simulink model "Non_linear_simulation"  (R2020b)
settings: Solver=FixedStepAuto  StartTime=0.0  StopTime=10  FixedStep=.001  RelTol=1e-3  EnableMultiTasking=on
values from neighbouring files (symbols this model uses):
  alphaPlotHandle = plot(inf,inf,'-b','linewidth',2)    [initialiseVisualiser.m]
  armPartPatchHandle = patch(Xt,Yt,Zt,C,'Edgecolor', edgecolor,'facealpha',facealpha,'clipping','off')    [initialiseVisualiser.m]
  armPartVertices = [X(:) Y(:) Z(:) ones(length(X(:)),1)]'    [initialiseVisualiser.m]
  drivePartPatchHandle = patch(Xt,Yt,Zt,C,'Edgecolor', edgecolor,'facealpha',facealpha,'clipping','off')    [initialiseVisualiser.m]
  drivePartVertices = [X(:) Y(:) Z(:) ones(length(X(:)),1)]'    [initialiseVisualiser.m]
  frameRate = 100    [AAP5_setup.m]
  pendPartPatchHandle = patch(Xt,Yt,Zt,C,'Edgecolor', edgecolor,'facealpha',facealpha,'clipping','off')    [initialiseVisualiser.m]
  pendPartVertices = [X(:) Y(:) Z(:) ones(length(X(:)),1)]'    [initialiseVisualiser.m]
  thetaPlotHandle = plot(inf,inf,'-r','linewidth',2)    [initialiseVisualiser.m]
settings Model: Creator=Dylan  LastModifiedBy=deniz
settings SolverCC: DecoupledContinuousIntegration=on
settings DataIOCC: LimitDataPoints=on  SaveFormat=StructureWithTime  ReturnWorkspaceOutputs=off
settings OptimizationCC: LifeSpan=inf
settings DebuggingCC: AllowSymbolicDim=off  SFUnexpectedBacktrackingDiag=warning  SFNoUnconditionalDefaultTransitionDiag=warning  SFExecutionAtInitializationDiag=none  ArithmeticOperatorsInVariantConditions=warning
settings HardwareCC: ProdBitPerSizeT=32  ProdBitPerPtrDiffT=32  ProdWordSize=32  ProdHWDeviceType=Specified
settings ModelReferenceCC: PropagateSignalLabelsOutOfModel=off
settings SFSimCC: SimUseLocalCustomCode=off  CustomCodeUndefinedFunction=UseInterfaceOnly  SimTargetLang=C++  GPUAcceleration=on  SimDLTargetLibrary=cudnn
settings RTWCC: RTWUseLocalCustomCode=off
settings CodeAppCC: StateflowObjectComments=on
settings GRTTargetCC: TargetLangStandard=C89/C90 (ANSI)
settings ConfigComp: CovMetricSettings=dw  CovSaveCumulativeToWorkspaceVar=on  CovSaveSingleToWorkspaceVar=on  CovExternalEMLEnable=off

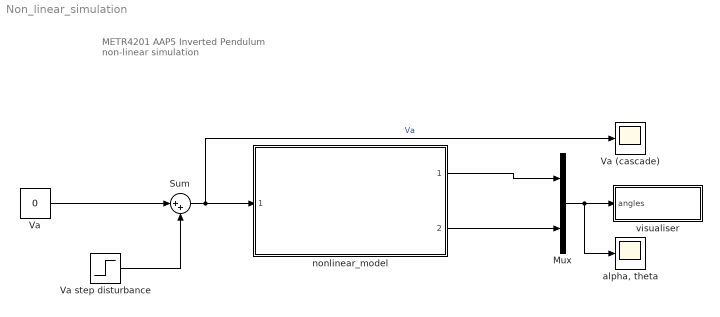
== system Non_linear_simulation ==
  note: METR4201 AAP5
      | Inverted Pendulum non-linear simulation
  Mux : Mux  Inputs=2
  Sum : Sum  Inputs=|++
  Va : Constant  Value=0
  Va (cascade) : Scope
  Va step disturbance : Step  SampleTime=0
  "alpha, theta" : Scope
  nonlinear_model : Subsystem  ReferencedSubsystem=nonlinear_model
      settings: MinAlgLoopOccurrences=on
  visualiser : Subsystem
  wires:
  Mux/1 -> "alpha, theta"/1, visualiser/1(angles)
  nonlinear_model/2 -> Mux/2
  nonlinear_model/1 -> Mux/1
  Sum/1 -> Va (cascade)/1, nonlinear_model/1  "Va"
  Va step disturbance/1 -> Sum/2
  Va/1 -> Sum/1

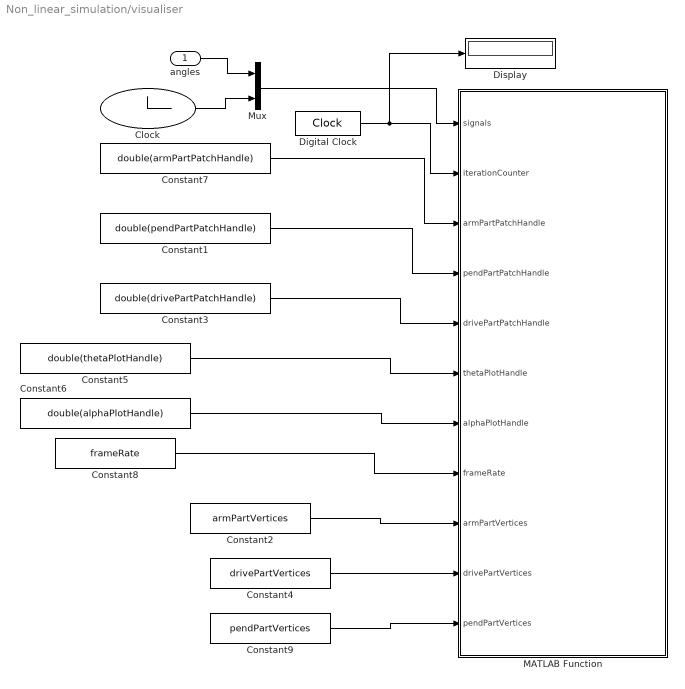
== system Non_linear_simulation/visualiser ==
  angles : Inport
  Clock : Clock
  Constant1 : Constant  Value=double(pendPartPatchHandle)
  Constant2 : Constant  Value=armPartVertices  VectorParams1D=off
  Constant3 : Constant  Value=double(drivePartPatchHandle)
  Constant4 : Constant  Value=drivePartVertices  VectorParams1D=off
  Constant5 : Constant  Value=double(thetaPlotHandle)
  Constant6 : Constant  Value=double(alphaPlotHandle)
  Constant7 : Constant  Value=double(armPartPatchHandle)
  Constant8 : Constant  Value=frameRate  VectorParams1D=off
  Constant9 : Constant  Value=pendPartVertices  VectorParams1D=off
  Digital Clock : DigitalClock  SampleTime=.001
  Display : Display
  MATLAB Function : MATLAB Function  TreatAsAtomicUnit=on
  Mux : Mux  Inputs=2
  wires:
  angles/1 -> Mux/1
  Mux/1 -> MATLAB Function/1(signals)
  Clock/1 -> Mux/2
  Constant7/1 -> MATLAB Function/3(armPartPatchHandle)
  Constant1/1 -> MATLAB Function/4(pendPartPatchHandle)
  Constant6/1 -> MATLAB Function/7(alphaPlotHandle)
  Constant5/1 -> MATLAB Function/6(thetaPlotHandle)
  Constant3/1 -> MATLAB Function/5(drivePartPatchHandle)
  Digital Clock/1 -> Display/1, MATLAB Function/2(iterationCounter)
  Constant8/1 -> MATLAB Function/8(frameRate)
  Constant2/1 -> MATLAB Function/9(armPartVertices)
  Constant4/1 -> MATLAB Function/10(drivePartVertices)
  Constant9/1 -> MATLAB Function/11(pendPartVertices)

== matlab function Non_linear_simulation/visualiser/MATLAB Function ==
  data: signals input; iterationCounter input; armPartPatchHandle input; pendPartPatchHandle input; drivePartPatchHandle input; thetaPlotHandle input; alphaPlotHandle input; frameRate input; armPartVertices input; drivePartVertices input; pendPartVertices input
function  updateVisualiser(signals, iterationCounter, armPartPatchHandle, pendPartPatchHandle, drivePartPatchHandle, thetaPlotHandle, alphaPlotHandle, frameRate, armPartVertices,drivePartVertices,pendPartVertices)

%
% We need the set and get functions for changing plots.
%
coder.extrinsic('set');
coder.extrinsic('get');
%
% Clear the theta and alpha plots if this is the first iteration.
%
if iterationCounter == 0
    set(thetaPlotHandle,'xData',inf,'yData',inf);
    set(alphaPlotHandle,'xData',inf,'yData',inf);

end

%
% Only update figure on every 2nd iteration.
%
if mod(iterationCounter,0.005) == 0
    
    alphaAngle = signals(1);
    thetaAngle = signals(2);
    currentTime = signals(3);
    
    %
    % New frame transformations.
    %
    BaseToArm = homogeneous_func(0,0,thetaAngle,0,0,12e-2);
    ArmToPendulum = homogeneous_func(alphaAngle,0,0,14.2e-2,0,5e-2);
    BaseToDrive = homogeneous_func(0,0,(-thetaAngle*5),0,0.036,12e-2);
    
    %
    % Update arm parts.
    %
    armPart_vertices_G_frame = BaseToArm * armPartVertices;
    Xt = reshape(armPart_vertices_G_frame(1,:),3,[]);
    Yt = reshape(armPart_vertices_G_frame(2,:),3,[]);
    Zt = reshape(armPart_vertices_G_frame(3,:),3,[]);
    set(armPartPatchHandle, 'xData', Xt, 'yData', Yt, 'zData', Zt);
    
    %
    % Update pendulum parts.
    %
    pendPart_vertices_G_frame = BaseToArm * ArmToPendulum* pendPartVertices;
    Xt = reshape(pendPart_vertices_G_frame(1,:),3,[]);
    Yt = reshape(pendPart_vertices_G_frame(2,:),3,[]);
    Zt = reshape(pendPart_vertices_G_frame(3,:),3,[]);
    set(pendPartPatchHandle, 'xData', Xt, 'yData', Yt, 'zData', Zt);
    
    %
    % Update drive gear parts.
    %
    drivePart_vertices_G_frame = BaseToDrive* drivePartVertices;
    Xt = reshape(drivePart_vertices_G_frame(1,:),3,[]);
    Yt = reshape(drivePart_vertices_G_frame(2,:),3,[]);
    Zt = reshape(drivePart_vertices_G_frame(3,:),3,[]);
    set(drivePartPatchHandle, 'xData', Xt, 'yData', Yt, 'zData', Zt);
%     
    %
    % Update theta plot.
    %
    times = [get(thetaPlotHandle,'xData'), currentTime];
    thetaAngles = [get(thetaPlotHandle,'yData'), thetaAngle*180/pi];
    set(thetaPlotHandle,'xdata',times,'ydata',thetaAngles);
%     
    %
    % Update alpha plot.
    %
    times = [get(alphaPlotHandle,'xData'), currentTime];
    alphaAngles = [get(alphaPlotHandle,'yData'), alphaAngle*180/pi];
    set(alphaPlotHandle,'xdata',times,'ydata',alphaAngles);
end
end

function [T] = homogeneous_func(ROLL, PITCH, YAW, X, Y, Z)
cy=cos(YAW);
cp=cos(PITCH);
cr=cos(ROLL);
sp=sin(PITCH);
sr=sin(ROLL);
sy=sin(YAW);
T=[cy*cp, cy*sp*sr-sy*cr, cy*sp*cr+sy*sr, X; sy*cp, sy*sp*sr+cy*cr, sy*sp*cr-cy*sr, Y;
    -sp, cp*sr, cp*cr, Z; 0,0,0,1];
end
